simulink model "pende3"  (Simulink 6.1)
settings: Solver=ode45  StartTime=0.0  StopTime=100.0  RelTol=1e-4
libraries: cstblocks x10, simulink x6
settings Model: Creator=rana  LastModifiedBy=rana  ExtModeTrigMode=oneshot  ExtModeArmWhenConnect=off  ExtModeAutoUpdateStatusClock=off
settings DataIOCC: LimitDataPoints=off
settings OptimizationCC: BlockReduction=off  BooleanDataType=off
settings HardwareCC: TargetUnknown=on
settings GRTTargetCC: ModelReferenceCompliant=off  MatFileLogging=off

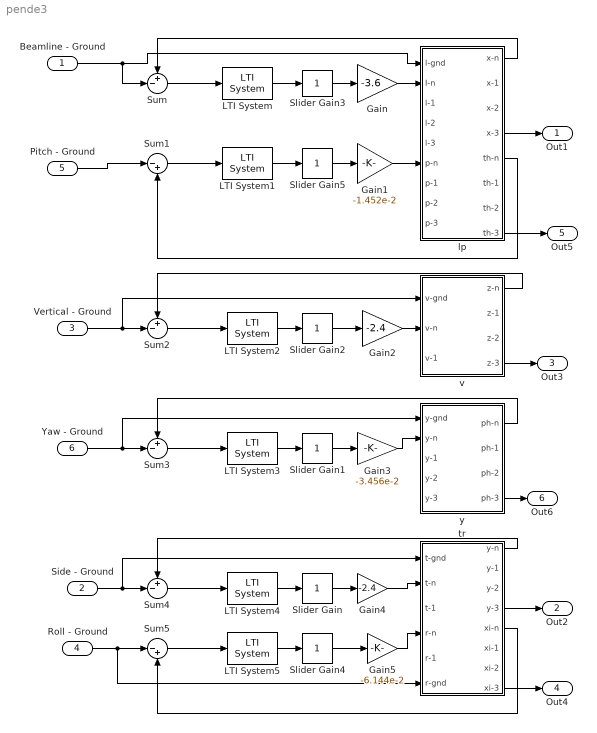
== system pende3 ==
  Beamline - Ground : Inport  Port=1  LatchInput=off
  Side - Ground : Inport  Port=2  LatchInput=off
  Vertical - Ground : Inport  Port=3  LatchInput=off
  Roll - Ground : Inport  Port=4  LatchInput=off
  Pitch - Ground : Inport  Port=5  LatchInput=off
  Yaw - Ground : Inport  Port=6  LatchInput=off
  Gain : Gain  Gain=-3.6
  Gain1 : Gain  Gain=-1.452e-2
  Gain2 : Gain  Gain=-2.4
  Gain3 : Gain  Gain=-3.456e-2
  Gain4 : Gain  Gain=-2.4
  Gain5 : Gain  Gain=-6.144e-2
  LTI System : cstblocks/LTI System  sys=ldamp  IC=0
  LTI System1 : cstblocks/LTI System  sys=pdamp  IC=0
  LTI System2 : cstblocks/LTI System  sys=vdamp  IC=0
  LTI System3 : cstblocks/LTI System  sys=ydamp  IC=0
  LTI System4 : cstblocks/LTI System  sys=tdamp  IC=0
  LTI System5 : cstblocks/LTI System  sys=rdamp  IC=0
  Slider Gain{,1..5} (6 alike) : simulink/Math Operations/Slider Gain  low=0  gain=1  high=2
  Sum{,2..4} (4 alike) : Sum  Inputs=+-|  InputSameDT=on
  Sum1 : Sum  Inputs=|-+  InputSameDT=on
  Sum5 : Sum  Inputs=|-+  InputSameDT=on
  lp : Subsystem
  tr : Subsystem
  v : Subsystem
  y : Subsystem
  Out1 : Outport
  Out2 : Outport  Port=2
  Out3 : Outport  Port=3
  Out4 : Outport  Port=4
  Out5 : Outport  Port=5
  Out6 : Outport  Port=6
  wires:
  Gain/1 -> lp/2(I-n)
  Gain2/1 -> v/2(v-n)
  Gain3/1 -> y/2(y-n)
  Gain4/1 -> tr/2(t-n)
  Gain5/1 -> tr/4(r-n)
  Gain1/1 -> lp/6(p-n)
  y/1(ph-n) -> Sum3/1
  tr/5(xi-n) -> Sum5/2
  tr/1(y-n) -> Sum4/1
  lp/5(th-n) -> Sum1/2
  lp/1(x-n) -> Sum/1
  Slider Gain1/1 -> Gain3/1
  Slider Gain2/1 -> Gain2/1
  Slider Gain/1 -> Gain4/1
  Slider Gain3/1 -> Gain/1
  Slider Gain5/1 -> Gain1/1
  Slider Gain4/1 -> Gain5/1
  LTI System/1 -> Slider Gain3/1
  LTI System2/1 -> Slider Gain2/1
  Sum1/1 -> LTI System1/1
  LTI System1/1 -> Slider Gain5/1
  LTI System3/1 -> Slider Gain1/1
  Sum3/1 -> LTI System3/1
  LTI System4/1 -> Slider Gain/1
  Sum4/1 -> LTI System4/1
  LTI System5/1 -> Slider Gain4/1
  Sum5/1 -> LTI System5/1
  v/1(z-n) -> Sum2/1
  Sum/1 -> LTI System/1
  Sum2/1 -> LTI System2/1
  Beamline - Ground/1 -> lp/1(l-gnd), Sum/2
  Pitch - Ground/1 -> Sum1/1
  Vertical - Ground/1 -> Sum2/2, v/1(v-gnd)
  Yaw - Ground/1 -> Sum3/2, y/1(y-gnd)
  Side - Ground/1 -> Sum4/2, tr/1(t-gnd)
  Roll - Ground/1 -> Sum5/1, tr/6(r-gnd)
  lp/4(x-3) -> Out1/1
  tr/4(y-3) -> Out2/1
  v/4(z-3) -> Out3/1
  tr/8(xi-3) -> Out4/1
  lp/8(th-3) -> Out5/1
  y/4(ph-3) -> Out6/1

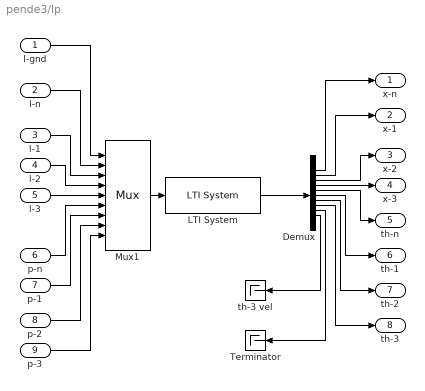
== system pende3/lp ==
  l-gnd : Inport  Port=1  LatchInput=off
  I-n : Inport  Port=2  LatchInput=off
  l-1 : Inport  Port=3  LatchInput=off
  l-2 : Inport  Port=4  LatchInput=off
  l-3 : Inport  Port=5  LatchInput=off
  p-n : Inport  Port=6  LatchInput=off
  p-1 : Inport  Port=7  LatchInput=off
  p-2 : Inport  Port=8  LatchInput=off
  p-3 : Inport  Port=9  LatchInput=off
  Demux : Demux  Outputs=10
  LTI System : cstblocks/LTI System  sys=lpe  IC=[0]
  Mux1 : Mux  Inputs=9
      settings: DisplayOption=signals
  Terminator : Terminator
  th-3 vel : Terminator
  x-n : Outport
  x-1 : Outport  Port=2
  x-2 : Outport  Port=3
  x-3 : Outport  Port=4
  th-n : Outport  Port=5
  th-1 : Outport  Port=6
  th-2 : Outport  Port=7
  th-3 : Outport  Port=8
  wires:
  Mux1/1 -> LTI System/1
  LTI System/1 -> Demux/1
  Demux/1 -> x-n/1
  Demux/2 -> x-1/1
  Demux/3 -> x-2/1
  Demux/4 -> x-3/1
  Demux/5 -> th-n/1
  Demux/6 -> th-1/1
  Demux/7 -> th-2/1
  Demux/8 -> th-3/1
  l-gnd/1 -> Mux1/1
  I-n/1 -> Mux1/2
  l-1/1 -> Mux1/3
  l-2/1 -> Mux1/4
  l-3/1 -> Mux1/5
  p-n/1 -> Mux1/6
  p-1/1 -> Mux1/7
  p-2/1 -> Mux1/8
  p-3/1 -> Mux1/9
  Demux/9 -> Terminator/1
  Demux/10 -> th-3 vel/1

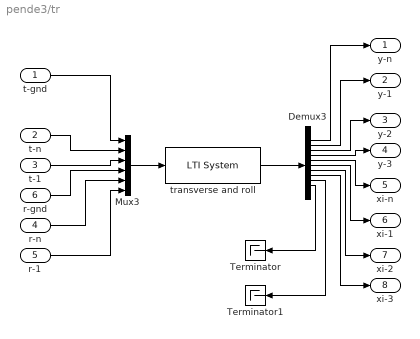
== system pende3/tr ==
  t-gnd : Inport  Port=1  LatchInput=off
  t-n : Inport  Port=2  LatchInput=off
  t-1 : Inport  Port=3  LatchInput=off
  r-n : Inport  Port=4  LatchInput=off
  r-1 : Inport  Port=5  LatchInput=off
  r-gnd : Inport  Port=6  LatchInput=off
  Demux3 : Demux  Outputs=10
  Mux3 : Mux  Inputs=6
  Terminator : Terminator
  Terminator1 : Terminator
  transverse and roll : cstblocks/LTI System  sys=trer  IC=[0]
  y-n : Outport
  y-1 : Outport  Port=2
  y-2 : Outport  Port=3
  y-3 : Outport  Port=4
  xi-n : Outport  Port=5
  xi-1 : Outport  Port=6
  xi-2 : Outport  Port=7
  xi-3 : Outport  Port=8
  wires:
  Mux3/1 -> transverse and roll/1
  transverse and roll/1 -> Demux3/1
  Demux3/1 -> y-n/1
  Demux3/2 -> y-1/1
  Demux3/3 -> y-2/1
  Demux3/4 -> y-3/1
  Demux3/5 -> xi-n/1
  Demux3/6 -> xi-1/1
  Demux3/7 -> xi-2/1
  Demux3/8 -> xi-3/1
  t-gnd/1 -> Mux3/1
  t-n/1 -> Mux3/2
  t-1/1 -> Mux3/3
  r-1/1 -> Mux3/6
  r-n/1 -> Mux3/5
  r-gnd/1 -> Mux3/4
  Demux3/9 -> Terminator1/1
  Demux3/10 -> Terminator/1

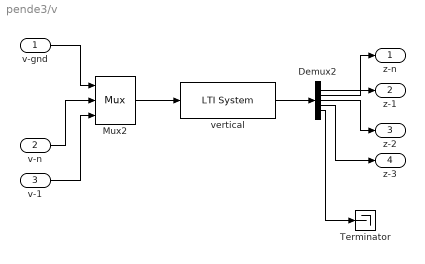
== system pende3/v ==
  v-gnd : Inport  Port=1  LatchInput=off
  v-n : Inport  Port=2  LatchInput=off
  v-1 : Inport  Port=3  LatchInput=off
  Demux2 : Demux  Outputs=5
  Mux2 : Mux  Inputs=3
      settings: DisplayOption=signals
  Terminator : Terminator
  vertical : cstblocks/LTI System  sys=ve  IC=[0]
  z-n : Outport
  z-1 : Outport  Port=2
  z-2 : Outport  Port=3
  z-3 : Outport  Port=4
  wires:
  Mux2/1 -> vertical/1
  vertical/1 -> Demux2/1
  v-gnd/1 -> Mux2/1
  Demux2/1 -> z-n/1
  Demux2/2 -> z-1/1
  Demux2/3 -> z-2/1
  Demux2/4 -> z-3/1
  v-1/1 -> Mux2/3
  v-n/1 -> Mux2/2
  Demux2/5 -> Terminator/1

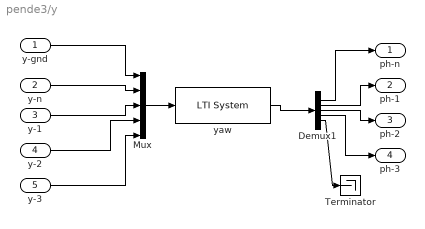
== system pende3/y ==
  y-gnd : Inport  Port=1  LatchInput=off
  y-n : Inport  Port=2  LatchInput=off
  y-1 : Inport  Port=3  LatchInput=off
  y-2 : Inport  Port=4  LatchInput=off
  y-3 : Inport  Port=5  LatchInput=off
  Demux1 : Demux  Outputs=5
  Mux : Mux  Inputs=5
  Terminator : Terminator
  yaw : cstblocks/LTI System  sys=ye  IC=[0]
  ph-n : Outport
  ph-1 : Outport  Port=2
  ph-2 : Outport  Port=3
  ph-3 : Outport  Port=4
  wires:
  y-gnd/1 -> Mux/1
  Mux/1 -> yaw/1
  yaw/1 -> Demux1/1
  Demux1/1 -> ph-n/1
  Demux1/2 -> ph-1/1
  Demux1/3 -> ph-2/1
  Demux1/4 -> ph-3/1
  y-3/1 -> Mux/5
  y-2/1 -> Mux/4
  y-1/1 -> Mux/3
  y-n/1 -> Mux/2
  Demux1/5 -> Terminator/1
